simulink model "LQR_Ref_Track_Const_Vx_Cf_Cr_SimContinous_5States"  (R2018a)
settings: Solver=FixedStepAuto  StartTime=0.0  StopTime=82  FixedStep=T  RelTol=1e-3
values from neighbouring files (symbols this model uses):
  A = [a11 a12 a13 ... (first row only)    [LQR_Ref_Track_Const_Vx_Cf_Cr_LinMod_3_state.m]    (also in LQR_Ref_Track_Const_Vx_Cf_Cr_LinMod_5_state.m = [0 1 0 0 0; 0 a11 0 a12 0; linearVehicleModel.m; linearVehicleModel2.m; vehicleDeviationModel.m = [0  1  0  0 0)
  B = [b1;b2;b3]    [LQR_Ref_Track_Const_Vx_Cf_Cr_LinMod_3_state.m]    (also in LQR_Ref_Track_Const_Vx_Cf_Cr_LinMod_5_state.m = [0;b1;0;b2;b3]; linearVehicleModel.m; linearVehicleModel2.m; vehicleDeviationModel.m = [0;b1;0;b2;b3])
  C = [0 1 0]    [LQR_Ref_Track_Const_Vx_Cf_Cr_LinMod_3_state.m]    (also in LQR_Ref_Track_Const_Vx_Cf_Cr_LinMod_5_state.m = [1 0 0 0 0; 0 0 0 1 0]; linearVehicleModel.m = eye(3,3); linearVehicleModel2.m = eye(3,3); vehicleDeviationModel.m = eye(5,5))
  K_lqi = lqi(sys,Q,R)    [LQR_Ref_Track_Const_Vx_Cf_Cr_LinMod_3_state.m]    (also in LQR_Ref_Track_Const_Vx_Cf_Cr_LinMod_5_state.m)
  Kc_lqr = Kc(1:3)    [LQR_Ref_Track_Const_Vx_Cf_Cr_LinMod_3_state.m]
  Kic = Kc(4)    [LQR_Ref_Track_Const_Vx_Cf_Cr_LinMod_3_state.m]
undefined symbols (not defined in the file or in its folder): Kc, sigbuilder_block
libraries: simulink_extras x1
settings Model: Creator=Shouvik Chakraborty  LastModifiedBy=Shouvik Chakraborty

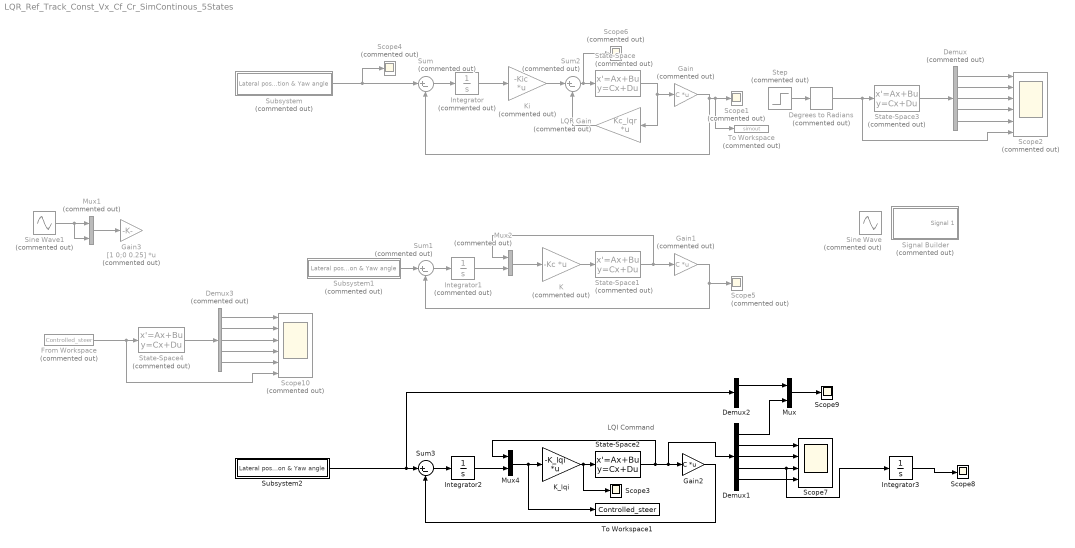
== system LQR_Ref_Track_Const_Vx_Cf_Cr_SimContinous_5States ==
  note: LQI Command
  Degrees to Radians : simulink_extras/Transformations/Degrees to Radians  Commented=on
  Demux : Demux  Commented=on  Outputs=5
  Demux1 : Demux  Outputs=5
  Demux2 : Demux  Outputs=2
  Demux3 : Demux  Commented=on  Outputs=5
  From Workspace : FromWorkspace  Commented=on  VariableName=Controlled_steer  SampleTime=0
  Gain : Gain  Commented=on  Gain=C  Multiplication=Matrix(K*u)
  Gain1 : Gain  Commented=on  Gain=C  Multiplication=Matrix(K*u)
  Gain2 : Gain  Gain=C  Multiplication=Matrix(K*u)
  Gain3 : Gain  Commented=on  Gain=[1 0;0 0.25]  Multiplication=Matrix(K*u)
  Integrator : Integrator  Commented=on
  Integrator1 : Integrator  Commented=on
  Integrator2 : Integrator
  Integrator3 : Integrator
  K : Gain  Commented=on  Gain=-Kc  Multiplication=Matrix(K*u)
  K_lqi : Gain  Gain=-K_lqi  Multiplication=Matrix(K*u)
  Ki : Gain  Commented=on  Gain=-Kic  Multiplication=Matrix(K*u)
  LQR Gain : Gain  Commented=on  Gain=Kc_lqr  Multiplication=Matrix(K*u)
  Mux : Mux  Inputs=2
  Mux1 : Mux  Commented=on  Inputs=2
  Mux2 : Mux  Commented=on  Inputs=2
  Mux4 : Mux  Inputs=2
  Scope{1,4..6} (4 alike) : Scope  Commented=on
  Scope10 : Scope  Commented=on  NumInputPorts=6
  Scope2 : Scope  Commented=on  NumInputPorts=6
  Scope3 : Scope
  Scope7 : Scope  NumInputPorts=4
  Scope8 : Scope
  Scope9 : Scope
  Signal Builder : Subsystem  Tag=STV Subsys  Commented=on  LoadFcn=sigbuilder_block('load');  StartFcn=sigbuilder_block('start');  StopFcn=sigbuilder_block('stop');  ClipboardFcn=sigbuilder_block('clipboard');  mask(Sigbuilder block){tuvar=[0:10]}
      mask help: Simulink:masks:SigbuilderBlock_MD
      mask init:
      | if ~strcmp(get_param(bdroot(gcbh),'SimulationStatus'),'stopped') tuvar = sigbuilder_block('maskInit'); end
      settings: CopyFcn=sigbuilder_block('copy');  DeleteFcn=sigbuilder_block('delete');  ModelCloseFcn=sigbuilder_block('modelClose');  PreSaveFcn=sigbuilder_block('preSave');  PauseFcn=sigbuilder_block('pause');  ContinueFcn=sigbuilder_block('continue');  NameChangeFcn=sigbuilder_block('namechange');  OpenFcn=sigbuilder_block('open',[437.6 199.2 550.4 400 ]);  CloseFcn=sigbuilder_block('close');
      mask Display: plot(0, 0, 100, 100,[2, 2, 32, 32, 2], [68, 8, 8, 68, 68],[32, 2], [38, 38], [32, 19, 2],[53, 60, 44], [32, 17, 17, 2],[16, 16, 31, 31]);txt = getActiveGroup(gcbh);text(2, 100, txt,'verticalAlignment', 'top');
  Sine Wave : Sin  Commented=on  Amplitude=30  Frequency=0.5  SampleTime=0
  Sine Wave1 : Sin  Commented=on  SampleTime=0
  State-Space{,1,3..4} (4 alike) : StateSpace  Commented=on  A=A  B=B  C=eye(5,5)  D=[0; 0; 0; 0; 0]  InitialCondition=0
  State-Space2 : StateSpace  A=A  B=B  C=eye(5,5)  D=[0; 0; 0; 0; 0]  InitialCondition=0
  Step : Step  Commented=on  Time=0.2  After=30  SampleTime=0.1
  Subsystem : Subsystem  Commented=on
  Subsystem1 : Subsystem  Commented=on
  Subsystem2 : Subsystem
  Sum : Sum  Commented=on  Inputs=|+-
  Sum1 : Sum  Commented=on  Inputs=|+-
  Sum2 : Sum  Commented=on  Inputs=|+-
  Sum3 : Sum  Inputs=|+-
  To Workspace : ToWorkspace  Commented=on  VariableName=simout  SaveFormat=Timeseries  SampleTime=-1
  To Workspace1 : ToWorkspace  VariableName=Controlled_steer  SaveFormat=Timeseries  SampleTime=-1
  wires:
  Sum/1 -> Integrator/1
  Integrator/1 -> Ki/1
  Sum2/1 -> Scope6/1, State-Space/1
  State-Space/1 -> Gain/1, LQR Gain/1
  LQR Gain/1 -> Sum2/2
  Subsystem/1(Lateral position & Yaw angle) -> Scope4/1, Sum/1
  Ki/1 -> Sum2/1
  Gain/1 -> To Workspace/1, Scope1/1, Sum/2
  Gain1/1 -> Scope5/1, Sum1/2
  State-Space1/1 -> Gain1/1, Mux2/1
  Subsystem1/1(Lateral position & Yaw angle) -> Sum1/1
  K/1 -> State-Space1/1
  Sum1/1 -> Integrator1/1
  Integrator1/1 -> Mux2/2
  Mux2/1 -> K/1
  Mux4/1 -> To Workspace1/1, K_lqi/1
  State-Space2/1 -> Demux1/1, Gain2/1, Mux4/1
  Sum3/1 -> Integrator2/1
  K_lqi/1 -> Scope3/1, State-Space2/1
  Gain2/1 -> Sum3/2
  Integrator2/1 -> Mux4/2
  Degrees to Radians/1 -> Scope2/6, State-Space3/1
  Demux/5 -> Scope2/5
  Demux/4 -> Scope2/4
  Demux/3 -> Scope2/3
  Demux/2 -> Scope2/2
  Demux/1 -> Scope2/1
  State-Space3/1 -> Demux/1
  Step/1 -> Degrees to Radians/1
  Subsystem2/1(Lateral position & Yaw angle) -> Demux2/1, Sum3/1
  Demux2/1 -> Mux/1
  Demux1/1 -> Mux/2
  Mux/1 -> Scope9/1
  Demux1/2 -> Scope7/1
  Demux1/3 -> Scope7/2
  Demux1/4 -> Integrator3/1, Scope7/3
  Demux1/5 -> Scope7/4
  Integrator3/1 -> Scope8/1
  Mux1/1 -> Gain3/1
  Sine Wave1/1 -> Mux1/2, Mux1/1
  Demux3/2 -> Scope10/2
  Demux3/4 -> Scope10/4
  Demux3/1 -> Scope10/1
  From Workspace/1 -> Scope10/6, State-Space4/1
  State-Space4/1 -> Demux3/1
  Demux3/5 -> Scope10/5
  Demux3/3 -> Scope10/3

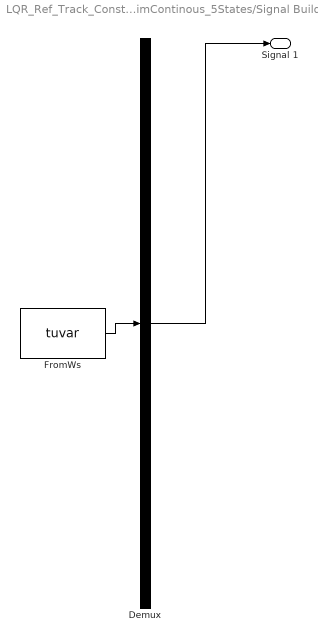
== system LQR_Ref_Track_Const_Vx_Cf_Cr_SimContinous_5States/Signal Builder ==
  Demux : Demux  Tag=STV Demux  Outputs=1
  FromWs : FromWorkspace  Tag=STV FromWs  VariableName=tuvar  SampleTime=0
      SigBuilderData=|
      | common.afterFinalStr = 'Extrapolate'
      | common.sampleTime = 0
      | dataSet.timeRange = [0 10]
      | dataSet.name = 'Group 1'
      | sbobj.Groups.Name = 'Group 1'
      | sbobj.Groups.Signals.Name = 'Signal 1'
      | sbobj.Groups.Signals.XData = [0 4 6 10]
      | sbobj.Groups.Signals.YData = [0 1 1 0]
  Signal 1 : Outport  Tag=STV Outport
  wires:
  Demux/1 -> Signal 1/1
  FromWs/1 -> Demux/1

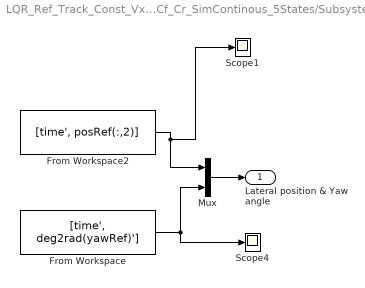
== system LQR_Ref_Track_Const_Vx_Cf_Cr_SimContinous_5States/Subsystem ==
  From Workspace : FromWorkspace  VariableName=[time', deg2rad(yawRef)']  SampleTime=0.1
  From Workspace2 : FromWorkspace  VariableName=[time', posRef(:,2)]  SampleTime=0.1
  Mux : Mux  Inputs=2
  Scope1 : Scope
  Scope4 : Scope
  Lateral position & Yaw angle : Outport
  wires:
  From Workspace/1 -> Scope4/1, Mux/2
  From Workspace2/1 -> Scope1/1, Mux/1
  Mux/1 -> Lateral position & Yaw angle/1

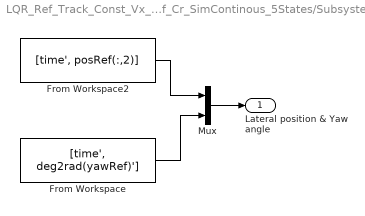
== system LQR_Ref_Track_Const_Vx_Cf_Cr_SimContinous_5States/Subsystem1 ==
  From Workspace : FromWorkspace  VariableName=[time', deg2rad(yawRef)']  SampleTime=0.1
  From Workspace2 : FromWorkspace  VariableName=[time', posRef(:,2)]  SampleTime=0.1
  Mux : Mux  Inputs=2
  Lateral position & Yaw angle : Outport
  wires:
  From Workspace/1 -> Mux/2
  From Workspace2/1 -> Mux/1
  Mux/1 -> Lateral position & Yaw angle/1

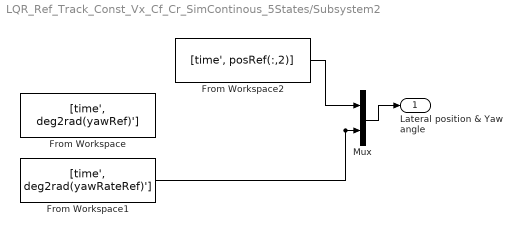
== system LQR_Ref_Track_Const_Vx_Cf_Cr_SimContinous_5States/Subsystem2 ==
  From Workspace : FromWorkspace  VariableName=[time', deg2rad(yawRef)']  SampleTime=0.1
  From Workspace1 : FromWorkspace  VariableName=[time', deg2rad(yawRateRef)']  SampleTime=0.1
  From Workspace2 : FromWorkspace  VariableName=[time', posRef(:,2)]  SampleTime=0.1
  Mux : Mux  Inputs=2
  Lateral position & Yaw angle : Outport
  wires:
  From Workspace2/1 -> Mux/1
  Mux/1 -> Lateral position & Yaw angle/1
  From Workspace1/1 -> Mux/2
